simulink model "Project_LQR"  (Simulink 9.1)
settings: Solver=VariableStepAuto  StartTime=0.0  StopTime=10.0  RelTol=1e-3
values from neighbouring files (symbols this model uses):
  A = [-0.0075 0; 0 -0.015]    [MODEL_PARAMETER_PROJECT.m]
  B = [1 1; -22.33 44.66]    [MODEL_PARAMETER_PROJECT.m]
  C = [1 0; 0 1]    [MODEL_PARAMETER_PROJECT.m]
  D = [0 0; 0 0]    [MODEL_PARAMETER_PROJECT.m]
undefined symbols (not defined in the file or in its folder): K
settings Model: SuppressorTable=22 serialization::archive 11 0 6 0 0 0 0 0  Creator=maclapuser  LastModifiedBy=maclapuser
settings DataIOCC: SaveFormat=Dataset
settings OptimizationCC: LifeSpan=auto
settings DebuggingCC: UnderspecifiedInitializationDetection=Simplified  MergeDetectMultiDrivingBlocksExec=error  SFUnexpectedBacktrackingDiag=error  SFNoUnconditionalDefaultTransitionDiag=error  SFExecutionAtInitializationDiag=warning
settings HardwareCC: ProdBitPerPointer=64  ProdBitPerSizeT=64  ProdBitPerPtrDiffT=64  ProdLargestAtomicFloat=Float  ProdIntDivRoundTo=Zero  ProdEndianess=LittleEndian  ProdWordSize=64  ProdHWDeviceType=Intel->x86-64 (Windows64)
settings ModelReferenceCC: PropagateSignalLabelsOutOfModel=on
settings CodeAppCC: StateflowObjectComments=off
settings GRTTargetCC: TargetLangStandard=C99 (ISO)  CombineOutputUpdateFcns=on  GRTInterface=off
settings ConfigComp: CovMetricSettings=dwe  CovHtmlReporting=off  CovSaveCumulativeToWorkspaceVar=off  CovSaveSingleToWorkspaceVar=off  CovExternalEMLEnable=on

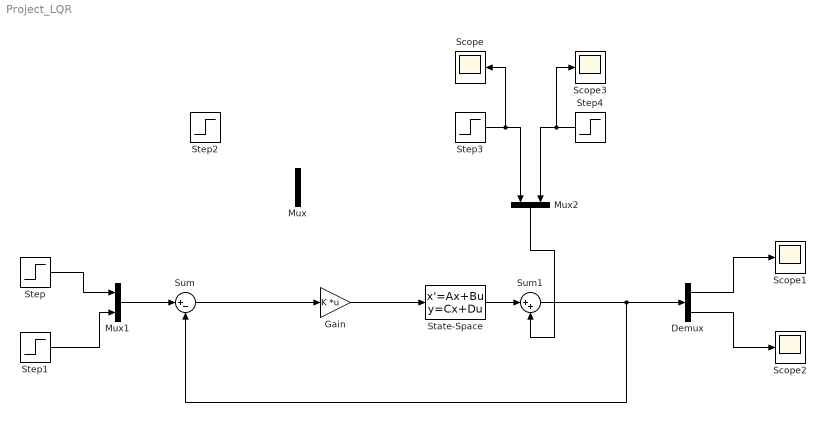
== system Project_LQR ==
  Demux : Demux  Outputs=2
  Gain : Gain  Gain=K  Multiplication=Matrix(K*u)
  Mux : Mux  Inputs=2
  Mux1 : Mux  Inputs=2
  Mux2 : Mux  Inputs=2
  Scope{,1..3} (4 alike) : Scope
  State-Space : StateSpace  A=A  B=B  C=C  D=D  InitialCondition="[0.1  0.1]"
  Step : Step  After=0  SampleTime=0
  Step1 : Step  After=0  SampleTime=0
  Step2 : Step  SampleTime=0
  Step3 : Step  Time=0.1  After=0  SampleTime=0
  Step4 : Step  Time=0.1  After=0  SampleTime=0
  Sum : Sum  Inputs=|+-
  Sum1 : Sum  Inputs=|++
  wires:
  Step/1 -> Mux1/1
  Step1/1 -> Mux1/2
  Mux1/1 -> Sum/1
  Sum/1 -> Gain/1
  Gain/1 -> State-Space/1
  Demux/1 -> Scope1/1
  Demux/2 -> Scope2/1
  Step4/1 -> Scope3/1, Mux2/2
  Step3/1 -> Scope/1, Mux2/1
  Mux2/1 -> Sum1/2
  Sum1/1 -> Sum/2, Demux/1
  State-Space/1 -> Sum1/1
